simulink model "V2021_M3_P1"  (R2021a)
settings: Solver=VariableStepAuto  StartTime=0.0  StopTime=10.0  RelTol=1e-3
values from neighbouring files (symbols this model uses):
  f_eff = 0.001 + (0.001 * NRP)    [M3_Script_Improved.m]
  J_eff = 0.00004 + (0.00001 * NRP)    [M3_Script_Improved.m]
  Kb = 0.02 + (0.001 * NRP)    [M3_Script_Improved.m]
  Kd = [0, 0, 0]    [M3_Script_Improved.m]
  Ki = [0, 0, 0]    [M3_Script_Improved.m]
  Kp = [0, 0, 0]    [M3_Script_Improved.m]
  Ktn = 0.026 + (0.001 * NRP)    [M3_Script_Improved.m]
  L = 0.062    [M3_Script_Improved.m]
  Lengan = 5.3    [M3_Script_Improved.m]
  Pos_ref = pos_ref_values(i)    [M3_Script_Improved.m]
  R = 2.5    [M3_Script_Improved.m]
libraries: simulink x1
settings Model: Creator=azzam  LastModifiedBy=azzam
settings DebuggingCC: UnconnectedInputMsg=none  UnconnectedOutputMsg=none  UnconnectedLineMsg=none
settings ModelReferenceCC: EnableRefExpFcnMdlSchedulingChecks=off
settings RTWCC: Description=Generic Real-Time Target  DLArmComputeVersion=20.02.1

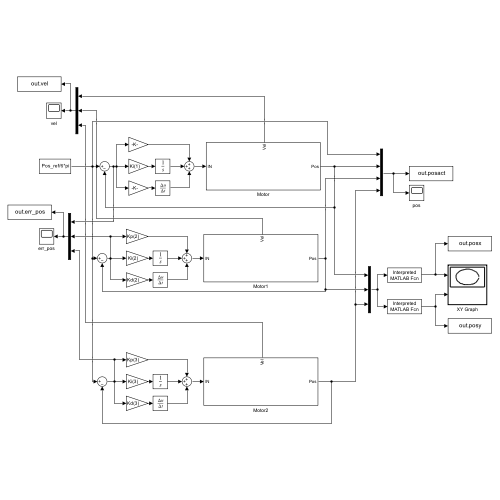
[thumbnail: Simulink's stored preview of the top-level diagram]
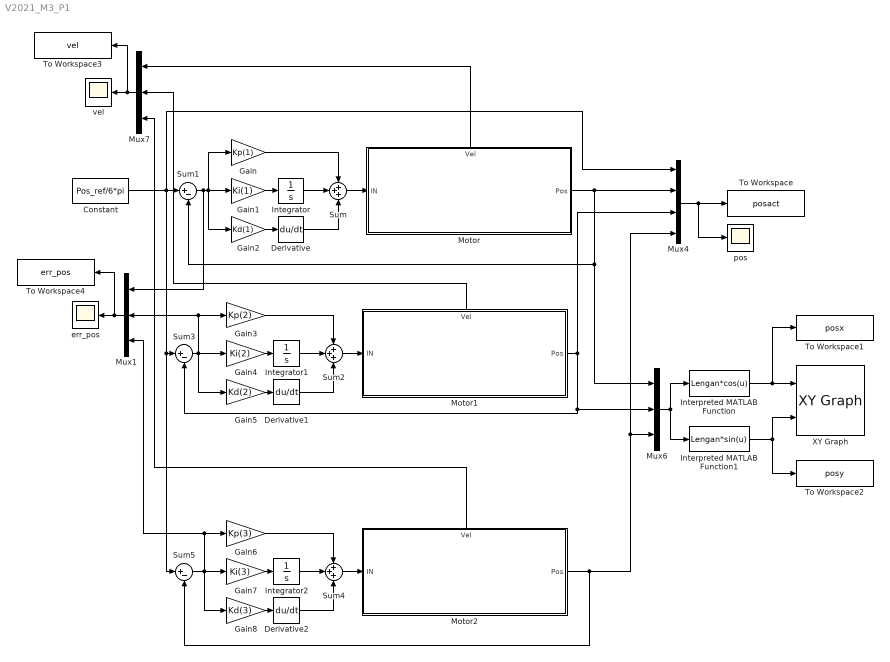
== system V2021_M3_P1 ==
  Constant : Constant  Value=Pos_ref/6*pi
  Derivative : Derivative
  Derivative1 : Derivative
  Derivative2 : Derivative
  Gain : Gain  Gain=Kp(1)
  Gain1 : Gain  Gain=Ki(1)
  Gain2 : Gain  Gain=Kd(1)
  Gain3 : Gain  Gain=Kp(2)
  Gain4 : Gain  Gain=Ki(2)
  Gain5 : Gain  Gain=Kd(2)
  Gain6 : Gain  Gain=Kp(3)
  Gain7 : Gain  Gain=Ki(3)
  Gain8 : Gain  Gain=Kd(3)
  Integrator : Integrator
  Integrator1 : Integrator
  Integrator2 : Integrator
  Interpreted MATLAB Function : MATLABFcn  MATLABFcn=Lengan*cos(u)
  Interpreted MATLAB Function1 : MATLABFcn  MATLABFcn=Lengan*sin(u)
  Motor : Subsystem
      settings: PortSchema="{\"entries\":[{\"content\":{\"sides\":[{\"content\":{\"connectorIds\":[\"In1\"]},\"type\":\"ConnectorPlacement.EquallySpacedRectSide\",\"uuid\":\"5d592437-2b24-436e-b414-64ae35424ef6\"},{\"content\":{\"connectorIds\":[\"Out1\"],\"side\":\"RIGHT\"},\"type\":\"ConnectorPlacement.EquallySpacedRectSide\",\"uuid\":\"34c7363f-afa0-43a5-b74e-2e83f8bd64af\"},{\"content\":{\"connectorIds\":[\"Out2\"],\"side\":\"TOP\"},\"type\":\"ConnectorPlacement.EquallySpacedRectSide\",\"uuid\":\"43639866-ebfc-48f9-acd8-6e486e6a6df9\"},{\"content\":{\"side\":\"BOTTOM\"},\"type\":\"ConnectorPlacement.EquallySpacedRectSide\",\"uuid\":\"e9d7ad21-e58b-4e41-ba70-2eed7a1b7de7\"}]},\"type\":\"ConnectorPlacement.EquallySpacedConnector\",\"uuid\":\"d37a131f-e295-4407-b67c-888faeed6def\"}],\"packageUris\":[\"http://schema.mathworks.com/mf0/Connector/R2020b\"],\"version\":\"1.0\"}"
  Motor1 : Subsystem
      settings: PortSchema="{\"entries\":[{\"content\":{\"sides\":[{\"content\":{\"connectorIds\":[\"In1\"]},\"type\":\"ConnectorPlacement.EquallySpacedRectSide\",\"uuid\":\"5d592437-2b24-436e-b414-64ae35424ef6\"},{\"content\":{\"connectorIds\":[\"Out1\"],\"side\":\"RIGHT\"},\"type\":\"ConnectorPlacement.EquallySpacedRectSide\",\"uuid\":\"34c7363f-afa0-43a5-b74e-2e83f8bd64af\"},{\"content\":{\"connectorIds\":[\"Out2\"],\"side\":\"TOP\"},\"type\":\"ConnectorPlacement.EquallySpacedRectSide\",\"uuid\":\"43639866-ebfc-48f9-acd8-6e486e6a6df9\"},{\"content\":{\"side\":\"BOTTOM\"},\"type\":\"ConnectorPlacement.EquallySpacedRectSide\",\"uuid\":\"e9d7ad21-e58b-4e41-ba70-2eed7a1b7de7\"}]},\"type\":\"ConnectorPlacement.EquallySpacedConnector\",\"uuid\":\"d37a131f-e295-4407-b67c-888faeed6def\"}],\"packageUris\":[\"http://schema.mathworks.com/mf0/Connector/R2020b\"],\"version\":\"1.0\"}"
  Motor2 : Subsystem
      settings: PortSchema="{\"entries\":[{\"content\":{\"sides\":[{\"content\":{\"connectorIds\":[\"In1\"]},\"type\":\"ConnectorPlacement.EquallySpacedRectSide\",\"uuid\":\"5d592437-2b24-436e-b414-64ae35424ef6\"},{\"content\":{\"connectorIds\":[\"Out1\"],\"side\":\"RIGHT\"},\"type\":\"ConnectorPlacement.EquallySpacedRectSide\",\"uuid\":\"34c7363f-afa0-43a5-b74e-2e83f8bd64af\"},{\"content\":{\"connectorIds\":[\"Out2\"],\"side\":\"TOP\"},\"type\":\"ConnectorPlacement.EquallySpacedRectSide\",\"uuid\":\"43639866-ebfc-48f9-acd8-6e486e6a6df9\"},{\"content\":{\"side\":\"BOTTOM\"},\"type\":\"ConnectorPlacement.EquallySpacedRectSide\",\"uuid\":\"e9d7ad21-e58b-4e41-ba70-2eed7a1b7de7\"}]},\"type\":\"ConnectorPlacement.EquallySpacedConnector\",\"uuid\":\"d37a131f-e295-4407-b67c-888faeed6def\"}],\"packageUris\":[\"http://schema.mathworks.com/mf0/Connector/R2020b\"],\"version\":\"1.0\"}"
  Mux1 : Mux  Inputs=3
  Mux4 : Mux
  Mux6 : Mux  Inputs=3
  Mux7 : Mux  Inputs=3
  Sum : Sum  Inputs=+++
  Sum1 : Sum  Inputs=|+-
  Sum2 : Sum  Inputs=+++
  Sum3 : Sum  Inputs=|+-
  Sum4 : Sum  Inputs=+++
  Sum5 : Sum  Inputs=|+-
  To Workspace : ToWorkspace  VariableName=posact  SaveFormat=Timeseries  SampleTime=-1
  To Workspace1 : ToWorkspace  VariableName=posx  SampleTime=-1
      settings: Save2DSignal=2-D array (concatenate along first dimension)
  To Workspace2 : ToWorkspace  VariableName=posy  SampleTime=-1
      settings: Save2DSignal=2-D array (concatenate along first dimension)
  To Workspace3 : ToWorkspace  VariableName=vel  SaveFormat=Timeseries  SampleTime=-1
  To Workspace4 : ToWorkspace  VariableName=err_pos  SaveFormat=Timeseries  SampleTime=-1
  XY Graph : simulink/Sinks/XY Graph  xmin=-1  xmax=1  ymin=-1  ymax=1  st=-1
  err_pos : Scope
  pos : Scope
  vel : Scope
  wires:
  Sum/1 -> Motor/1(IN)
  Integrator/1 -> Sum/2
  Gain2/1 -> Derivative/1
  Gain1/1 -> Integrator/1
  Derivative/1 -> Sum/3
  Gain/1 -> Sum/1
  Sum1/1 -> Mux1/1, Gain2/1, Gain/1, Gain1/1
  Mux7/1 -> To Workspace3/1, vel/1
  Constant/1 -> Sum3/1, Sum5/1, Mux4/1, Sum1/1
  Motor/2(Vel) -> Mux7/1
  Integrator1/1 -> Sum2/2
  Gain5/1 -> Derivative1/1
  Gain3/1 -> Sum2/1
  Gain4/1 -> Integrator1/1
  Sum3/1 -> Gain5/1, Mux1/2, Gain3/1, Gain4/1
  Derivative1/1 -> Sum2/3
  Sum2/1 -> Motor1/1(IN)
  Gain8/1 -> Derivative2/1
  Gain6/1 -> Sum4/1
  Integrator2/1 -> Sum4/2
  Sum4/1 -> Motor2/1(IN)
  Sum5/1 -> Mux1/3, Gain6/1, Gain8/1, Gain7/1
  Derivative2/1 -> Sum4/3
  Gain7/1 -> Integrator2/1
  Motor2/1(Pos) -> Sum5/2, Mux6/3, Mux4/4
  Motor1/1(Pos) -> Mux6/2, Sum3/2, Mux4/3
  Motor/1(Pos) -> Mux6/1, Sum1/2, Mux4/2
  Motor1/2(Vel) -> Mux7/2
  Motor2/2(Vel) -> Mux7/3
  Mux1/1 -> To Workspace4/1, err_pos/1
  Mux6/1 -> Interpreted MATLAB Function/1, Interpreted MATLAB Function1/1
  Interpreted MATLAB Function/1 -> To Workspace1/1, XY Graph/1
  Interpreted MATLAB Function1/1 -> XY Graph/2, To Workspace2/1
  Mux4/1 -> pos/1, To Workspace/1

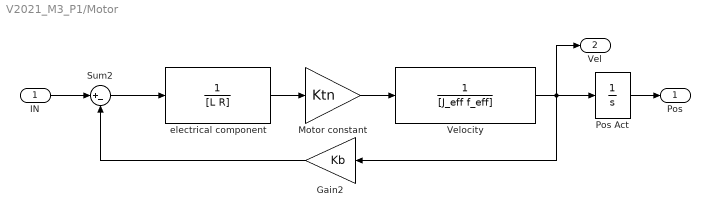
== system V2021_M3_P1/Motor ==
  IN : Inport
  Gain2 : Gain  Gain=Kb
  Motor constant : Gain  Gain=Ktn
  Pos Act : Integrator
  Sum2 : Sum  Inputs=|+-
  Velocity : TransferFcn  Denominator=[J_eff f_eff]
  electrical component : TransferFcn  Denominator=[L R]
  Pos : Outport
  Vel : Outport  Port=2
  wires:
  electrical component/1 -> Motor constant/1
  Motor constant/1 -> Velocity/1
  Sum2/1 -> electrical component/1
  IN/1 -> Sum2/1
  Gain2/1 -> Sum2/2
  Velocity/1 -> Vel/1, Pos Act/1, Gain2/1
  Pos Act/1 -> Pos/1

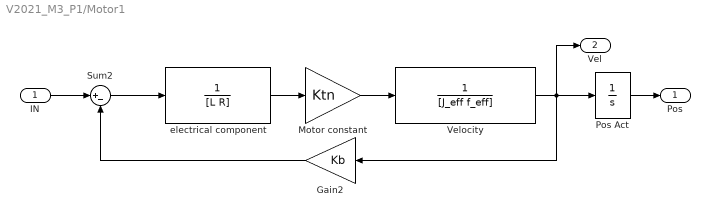
== system V2021_M3_P1/Motor1 ==
  IN : Inport
  Gain2 : Gain  Gain=Kb
  Motor constant : Gain  Gain=Ktn
  Pos Act : Integrator
  Sum2 : Sum  Inputs=|+-
  Velocity : TransferFcn  Denominator=[J_eff f_eff]
  electrical component : TransferFcn  Denominator=[L R]
  Pos : Outport
  Vel : Outport  Port=2
  wires:
  electrical component/1 -> Motor constant/1
  Motor constant/1 -> Velocity/1
  Sum2/1 -> electrical component/1
  IN/1 -> Sum2/1
  Gain2/1 -> Sum2/2
  Velocity/1 -> Vel/1, Pos Act/1, Gain2/1
  Pos Act/1 -> Pos/1

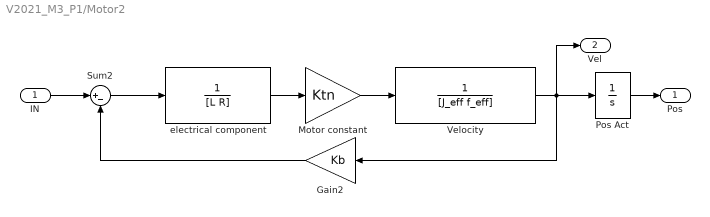
== system V2021_M3_P1/Motor2 ==
  IN : Inport
  Gain2 : Gain  Gain=Kb
  Motor constant : Gain  Gain=Ktn
  Pos Act : Integrator
  Sum2 : Sum  Inputs=|+-
  Velocity : TransferFcn  Denominator=[J_eff f_eff]
  electrical component : TransferFcn  Denominator=[L R]
  Pos : Outport
  Vel : Outport  Port=2
  wires:
  electrical component/1 -> Motor constant/1
  Motor constant/1 -> Velocity/1
  Sum2/1 -> electrical component/1
  IN/1 -> Sum2/1
  Gain2/1 -> Sum2/2
  Velocity/1 -> Vel/1, Pos Act/1, Gain2/1
  Pos Act/1 -> Pos/1
